simulink model "Feedback_ThreeLink"  (R2020b)
settings: Solver=VariableStepAuto  StartTime=0.0  StopTime=10.0  RelTol=1e-3
settings Model: Creator=MR.co  LastModifiedBy=MR.co

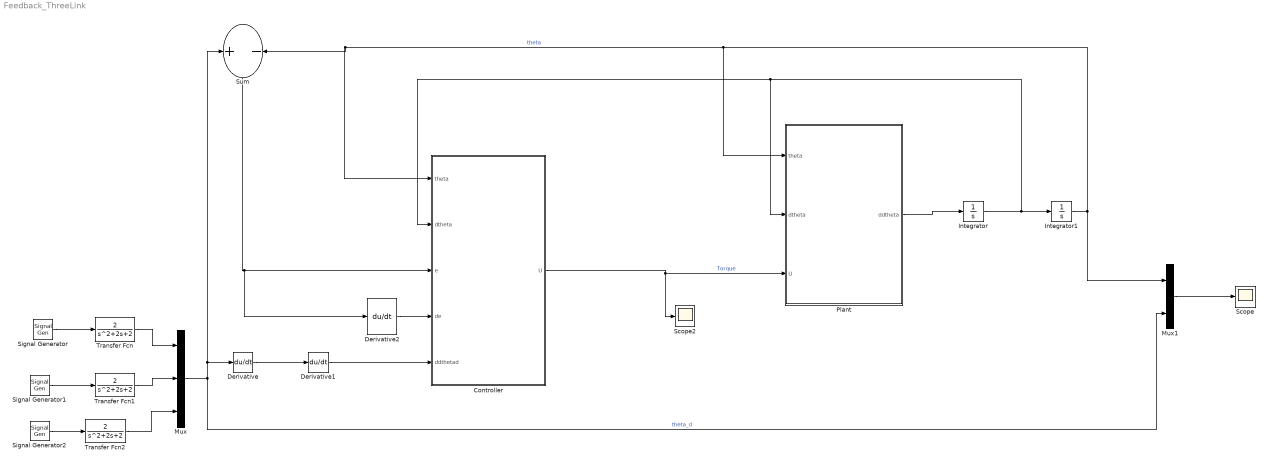
== system Feedback_ThreeLink ==
  Controller : MATLAB Function  TreatAsAtomicUnit=on
  Derivative : Derivative
  Derivative1 : Derivative
  Derivative2 : Derivative
  Integrator : Integrator  InitialCondition=zeros(3,1)
  Integrator1 : Integrator  InitialCondition=randn(3,1)
  Mux : Mux  Inputs=3
  Mux1 : Mux  Inputs=2
  Plant : MATLAB Function  TreatAsAtomicUnit=on
  Scope : Scope
  Scope2 : Scope
  Signal Generator : SignalGenerator  Amplitude=2  Frequency=pi  Units=rad/sec
  Signal Generator1 : SignalGenerator  WaveForm=square  Amplitude=3  Frequency=pi/2  Units=rad/sec
  Signal Generator2 : SignalGenerator  WaveForm=square  Frequency=pi/3  Units=rad/sec
  Sum : Sum  Inputs=+|-
  Transfer Fcn : TransferFcn  Numerator=[2]  Denominator=[1 2 2]
  Transfer Fcn1 : TransferFcn  Numerator=[2]  Denominator=[1 2 2]
  Transfer Fcn2 : TransferFcn  Numerator=[2]  Denominator=[1 2 2]
  wires:
  Signal Generator2/1 -> Transfer Fcn2/1
  Sum/1 -> Derivative2/1, Controller/3(e)
  Transfer Fcn2/1 -> Mux/3
  Transfer Fcn1/1 -> Mux/2
  Plant/1(ddtheta) -> Integrator/1
  Mux1/1 -> Scope/1
  Integrator/1 -> Plant/2(dtheta), Controller/2(dtheta), Integrator1/1
  Controller/1(U) -> Scope2/1, Plant/3(U)  "Torque"
  Derivative1/1 -> Controller/5(ddthetad)
  Integrator1/1 -> Plant/1(theta), Sum/2, Controller/1(theta), Mux1/1  "theta"
  Signal Generator1/1 -> Transfer Fcn1/1
  Transfer Fcn/1 -> Mux/1
  Derivative/1 -> Derivative1/1
  Derivative2/1 -> Controller/4(de)
  Signal Generator/1 -> Transfer Fcn/1
  Mux/1 -> Sum/1, Derivative/1, Mux1/2  "theta_d"

== matlab function Feedback_ThreeLink/Controller ==
  data: theta input; U output; dtheta input; e input; de input; ddthetad input
function U = fcn( theta , dtheta , e , de, ddthetad)


    m1 = 1 ; %kg
    m2 = 1 ; %kg
    m3 = 1 ; %kg

    ac1 = .5 ; %m
    ac2 = .5 ; %m
    ac3 = .5 ; %m

    a1 = 1 ; %m
    a2 = 1 ; %m
    a3 = 1 ; %m

    I1 = 1/12 * m1 * a1^2 ; %kg.N
    I2 = 1/12 * m2 * a2^2 ; %kg.N
    I3 = 1/12 * m3 * a3^2 ; %kg.N

    g = 9.8; %m/s^2


    M = zeros(3,3) ;
    M(1,1) = I1+I2+I3+m1*ac1^2+m2*(a1^2+ac2^2+ 2*a1*ac2*cos(theta(2)))+m3*(a1^2+a2^2+ac3^2+2*a1*a2*cos(theta(2))+2*a1*ac3*cos(theta(2)+theta(3))+2*a2*ac3*cos(theta(3)) );
    M(1,2) = I2+I3 + m2*(ac2^2+a1*ac2*cos(theta(2)))+m3*(a2^2+ac3^2+a1*a2*cos(theta(2))+2*a2*ac3*cos(theta(3))+a1*ac3*cos(theta(2)+theta(3)) );
    M(2,1) = M(1,2) ;    
    M(3,1) = I3+m3*(ac3^2+a2*ac3*cos(theta(3))+a1*ac3*cos(theta(2)+theta(3)) );
    M(1,3) = M(3,1) ;
    M(3,2) = I3+m3*(ac3^2+a2*ac3*cos(theta(3))) ;
    M(2,3) = M(3,2) ;
    M(2,2) = I2+I3+m2*ac2^2+m3*((a2^2+ac3^2)+2*a2*ac3*cos(theta(3))) ;
    M(3,3) = I3+m3*ac3^2 ;

    B=zeros(3,1);

    B(1) = -m2*a1*ac2*(2*dtheta(1)+dtheta(2))*sin(theta(2))* dtheta(2)...
        -m3*(a1*a2*(2*dtheta(1)+dtheta(2))*sin(theta(2))+a1*ac3*(2*dtheta(1)+dtheta(2)+dtheta(3))*sin(theta(2)+theta(3))+a2*ac3*(2*dtheta(1)+dtheta(2)+dtheta(3))*sin(theta(3)));

    B(2) = -m2*(a1*ac2*((dtheta(1)^2)+dtheta(1)*dtheta(2))*sin(theta(2)) + a1*ac2*dtheta(1)*sin(theta(2))*dtheta(2))-...
        m3*(a1*a2*((dtheta(1)^2)+dtheta(1)*dtheta(2)) + a1*ac3*((dtheta(1)^2)+dtheta(1)*dtheta(2)+dtheta(1)*dtheta(3))*sin(theta(2)+theta(3)) + ...
        a2*ac3*((dtheta(1)^2)+2*dtheta(1)*dtheta(2)+dtheta(1)*dtheta(3)+(dtheta(2)^2)+dtheta(2)*dtheta(3))*sin(theta(3)) + ...
        a1*a2*dtheta(1)*sin(theta(2))*dtheta(2) + a1*ac3*dtheta(1)*dtheta(2)*sin(theta(2)+theta(3)) + ...
        a2*ac3*(2*dtheta(1)+2*dtheta(2)+dtheta(3))*sin(theta(3)));

    B(3) = -m3*(a1*ac3*((dtheta(1)^2)+dtheta(1)*dtheta(2)+dtheta(1)*dtheta(3))*sin(theta(2)+theta(3))+ ...
        a2*ac3*((dtheta(1)^2)+2*dtheta(1)*dtheta(2)+dtheta(1)*dtheta(3)+(dtheta(2)^2)+dtheta(2)*dtheta(3))*sin(theta(3)) + ...
        a1*ac3*dtheta(1)*dtheta(3)*sin(theta(2)+theta(3)) + ...
        a2*ac3*(dtheta(1)+dtheta(2))*sin(theta(3))*dtheta(3));

    G = zeros(3,1);

    G(1) = g * ( cos(theta(1)) * (m1 * ac1 + m2 * a1 + m3 * a1) + cos(theta(1)+theta(2)) * (m2 * ac2 + m3 * a2) + cos(theta(1) + theta(2) + theta(3)) * (m3 * ac3));
    G(2) = g * ((m2 * ac2 + m3 * a2) * cos(theta(1)+theta(2)) + m3 * ac3 * cos(theta(1) + theta(2) + theta(3)));
    G(3) = g *(m3 * ac3 * cos(theta(1) + theta(2) + theta(3)));

    k1 = 16 * eye(3);
    k2 = 64 * eye(3);
    v = ddthetad + k1 * de + k2 *e;

    U = M * v + B + G;

== matlab function Feedback_ThreeLink/Plant ==
  data: theta input; ddtheta output; dtheta input; U input
function ddtheta = fcn( theta , dtheta , U )


    m1 = 1 ; %kg
    m2 = 1 ; %kg
    m3 = 1 ; %kg

    ac1 = .5 ; %m
    ac2 = .5 ; %m
    ac3 = .5 ; %m

    a1 = 1 ; %m
    a2 = 1 ; %m
    a3 = 1 ; %m

    I1 = 1/12 * m1 * a1^2 ; %kg.N
    I2 = 1/12 * m2 * a2^2 ; %kg.N
    I3 = 1/12 * m3 * a3^2 ; %kg.N

    g = 9.8; %m/s^2


    M = zeros(3,3) ;
    M(1,1) = I1+I2+I3+m1*ac1^2+m2*(a1^2+ac2^2+ 2*a1*ac2*cos(theta(2)))+m3*(a1^2+a2^2+ac3^2+2*a1*a2*cos(theta(2))+2*a1*ac3*cos(theta(2)+theta(3))+2*a2*ac3*cos(theta(3)) );
    M(1,2) = I2+I3 + m2*(ac2^2+a1*ac2*cos(theta(2)))+m3*(a2^2+ac3^2+a1*a2*cos(theta(2))+2*a2*ac3*cos(theta(3))+a1*ac3*cos(theta(2)+theta(3)) );
    M(2,1) = M(1,2) ;    
    M(3,1) = I3+m3*(ac3^2+a2*ac3*cos(theta(3))+a1*ac3*cos(theta(2)+theta(3)) );
    M(1,3) = M(3,1) ;
    M(3,2) = I3+m3*(ac3^2+a2*ac3*cos(theta(3))) ;
    M(2,3) = M(3,2) ;
    M(2,2) = I2+I3+m2*ac2^2+m3*((a2^2+ac3^2)+2*a2*ac3*cos(theta(3))) ;
    M(3,3) = I3+m3*ac3^2 ;

    B=zeros(3,1);

    B(1) = -m2*a1*ac2*(2*dtheta(1)+dtheta(2))*sin(theta(2))* dtheta(2)...
        -m3*(a1*a2*(2*dtheta(1)+dtheta(2))*sin(theta(2))+a1*ac3*(2*dtheta(1)+dtheta(2)+dtheta(3))*sin(theta(2)+theta(3))+a2*ac3*(2*dtheta(1)+dtheta(2)+dtheta(3))*sin(theta(3)));

    B(2) = -m2*(a1*ac2*((dtheta(1)^2)+dtheta(1)*dtheta(2))*sin(theta(2)) + a1*ac2*dtheta(1)*sin(theta(2))*dtheta(2))-...
        m3*(a1*a2*((dtheta(1)^2)+dtheta(1)*dtheta(2)) + a1*ac3*((dtheta(1)^2)+dtheta(1)*dtheta(2)+dtheta(1)*dtheta(3))*sin(theta(2)+theta(3)) + ...
        a2*ac3*((dtheta(1)^2)+2*dtheta(1)*dtheta(2)+dtheta(1)*dtheta(3)+(dtheta(2)^2)+dtheta(2)*dtheta(3))*sin(theta(3)) + ...
        a1*a2*dtheta(1)*sin(theta(2))*dtheta(2) + a1*ac3*dtheta(1)*dtheta(2)*sin(theta(2)+theta(3)) + ...
        a2*ac3*(2*dtheta(1)+2*dtheta(2)+dtheta(3))*sin(theta(3)));

    B(3) = -m3*(a1*ac3*((dtheta(1)^2)+dtheta(1)*dtheta(2)+dtheta(1)*dtheta(3))*sin(theta(2)+theta(3))+ ...
        a2*ac3*((dtheta(1)^2)+2*dtheta(1)*dtheta(2)+dtheta(1)*dtheta(3)+(dtheta(2)^2)+dtheta(2)*dtheta(3))*sin(theta(3)) + ...
        a1*ac3*dtheta(1)*dtheta(3)*sin(theta(2)+theta(3)) + ...
        a2*ac3*(dtheta(1)+dtheta(2))*sin(theta(3))*dtheta(3));

    G = zeros(3,1);

    G(1) = g * ( cos(theta(1)) * (m1 * ac1 + m2 * a1 + m3 * a1) + cos(theta(1)+theta(2)) * (m2 * ac2 + m3 * a2) + cos(theta(1) + theta(2) + theta(3)) * (m3 * ac3));
    G(2) = g * ((m2 * ac2 + m3 * a2) * cos(theta(1)+theta(2)) + m3 * ac3 * cos(theta(1) + theta(2) + theta(3)));
    G(3) = g *(m3 * ac3 * cos(theta(1) + theta(2) + theta(3)));

    ddtheta = M\(U -B - G ) ;
